simulink model "zadanie_3"  (Simulink 7.7)
settings: Solver=ode4  StartTime=0.0  StopTime=20.0  FixedStep=0.01  RelTol=1e-3
values from neighbouring files (symbols this model uses):
  A = A_tab(i)    [lab4.m]    (also in zadania_3.m)
  a = a_tab(j)    [lab4.m]    (also in zadania_3.m)
  b = b_tab(j)    [lab4.m]    (also in zadania_3.m)
  w = w_tab(i)    [lab4.m]    (also in zadania_3.m)
settings Model: Creator=Aleksander  LastModifiedBy=Jacek
settings DataIOCC: LimitDataPoints=off  SignalLoggingSaveFormat=Dataset
settings OptimizationCC: ExpressionDepthLimit=128
settings CodeAppCC: CustomSymbolStrType=$N$R$M_T
settings GRTTargetCC: CombineOutputUpdateFcns=on

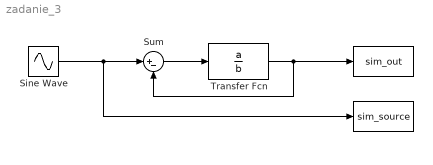
== system zadanie_3 ==
  " " : ToWorkspace  VariableName=sim_out  SampleTime=-1  SaveFormat=Array
  "  " : ToWorkspace  VariableName=sim_source  SampleTime=-1  SaveFormat=Array
  Sine Wave : Sin  Amplitude=A  Frequency=w  Phase=fi  SampleTime=0
  Sum : Sum  Inputs=|+-
  Transfer Fcn : TransferFcn  Numerator=a  Denominator=b
  wires:
  Sum/1 -> Transfer Fcn/1
  Transfer Fcn/1 -> Sum/2, " "/1
  Sine Wave/1 -> Sum/1, "  "/1
